simulink model "IAirHt_DD"  (R2016b)
settings: configuration reference "CodeGenConfigSet" (kept outside this file)
values from neighbouring files (symbols this model uses):
  IAirHt_stPsDiaDisbl_C = Calibration.Parameter    [init_IAirHt_DD.m]
  IAirHt_stPsDisbl_C = Calibration.Parameter    [init_IAirHt_DD.m]
  SigTst_stIAirHt_C = Calibration.Parameter    [init_IAirHt_DD.m]
  SigTst_swtIAirHt_C = Calibration.Parameter    [init_IAirHt_DD.m]
undefined symbols (not defined in the file or in its folder): Switch_conv
libraries: simulink x4
settings Model: Creator=Wei Liang  LastModifiedBy=liutao
settings ConfigSetRef: SourceLocation=Base Workspace

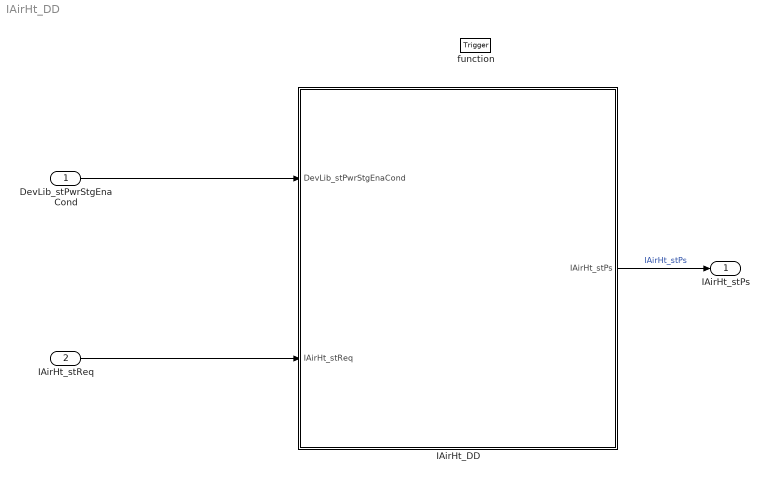
== system IAirHt_DD ==
  DevLib_stPwrStgEnaCond : Inport  Description=Control unit status relevant to power stage deactivation/error diagnosis  OutMin=0  OutMax=65535  OutDataTypeStr=State_uint16
  IAirHt_stReq : Inport  Description=Logical Output of Intake Air Heating  Port=2  OutMin=0  OutMax=1  OutDataTypeStr=boolean
  function : TriggerPort  TriggerType=function-call  VariantControl=Variant
  IAirHt_DD : Subsystem
  IAirHt_stPs : Outport  Description=Logical Output of Intake Air Heating  OutMin=0  OutMax=1  OutDataTypeStr=boolean
  wires:
  DevLib_stPwrStgEnaCond/1 -> IAirHt_DD/1(DevLib_stPwrStgEnaCond)
  IAirHt_stReq/1 -> IAirHt_DD/2(IAirHt_stReq)
  IAirHt_DD/1(IAirHt_stPs) -> IAirHt_stPs/1  "IAirHt_stPs"

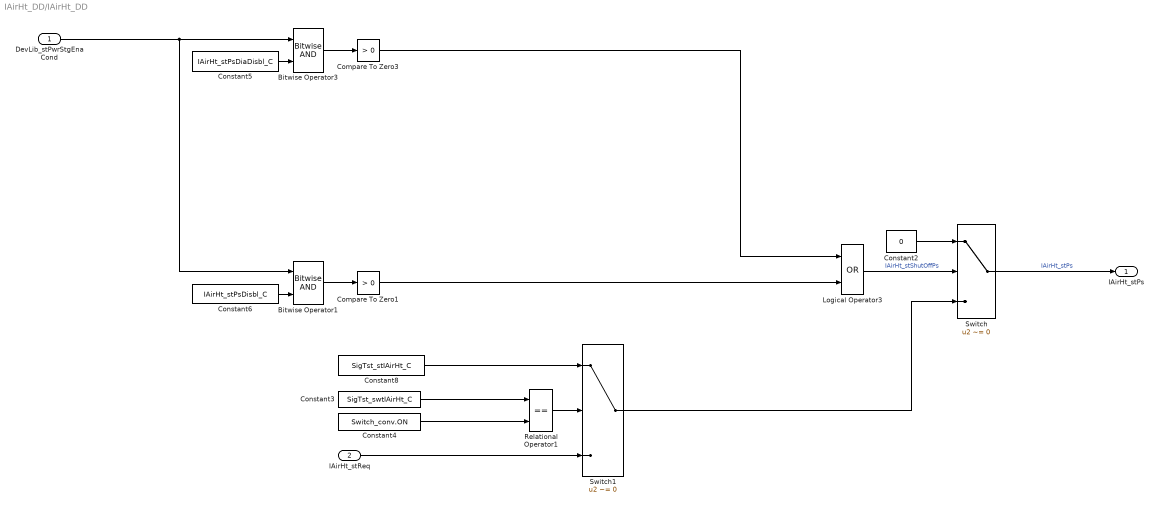
== system IAirHt_DD/IAirHt_DD ==
  DevLib_stPwrStgEnaCond : Inport  Description=Control unit status relevant to power stage deactivation/error diagnosis  OutMin=0  OutMax=65535  OutDataTypeStr=State_uint16
  IAirHt_stReq : Inport  Description=Logical Output of Intake Air Heating  Port=2  OutMin=0  OutMax=1  OutDataTypeStr=boolean
  Bitwise Operator1 : simulink/Logic and Bit Operations/Bitwise Operator  logicop=AND  UseBitMask=off  NumInputPorts=2  BitMask=bin2dec('00010000')  BitMaskRealWorld=Stored Integer
  Bitwise Operator3 : simulink/Logic and Bit Operations/Bitwise Operator  logicop=AND  UseBitMask=off  NumInputPorts=2  BitMask=bin2dec('00010000')  BitMaskRealWorld=Stored Integer
  Compare To Zero1 : simulink/Logic and Bit Operations/Compare To Zero  relop=>  OutDataTypeStr=uint8
  Compare To Zero3 : simulink/Logic and Bit Operations/Compare To Zero  relop=>  OutDataTypeStr=uint8
  Constant2 : Constant  Value=0  OutDataTypeStr=boolean  SampleTime=-1
  Constant3 : Constant  Value=SigTst_swtIAirHt_C
  Constant4 : Constant  Value=Switch_conv.ON
  Constant5 : Constant  Value=IAirHt_stPsDiaDisbl_C
  Constant6 : Constant  Value=IAirHt_stPsDisbl_C
  Constant8 : Constant  Value=SigTst_stIAirHt_C
  Logical Operator3 : Logic  Operator=OR  AllPortsSameDT=off  OutDataTypeStr=boolean
  Relational Operator1 : RelationalOperator  Operator===  OutDataTypeStr=boolean  RndMeth=Nearest
  Switch : Switch  Criteria=u2 ~= 0  SaturateOnIntegerOverflow=on  InputSameDT=on
  Switch1 : Switch  Criteria=u2 ~= 0  SaturateOnIntegerOverflow=on  InputSameDT=on
  IAirHt_stPs : Outport
  wires:
  Constant4/1 -> Relational Operator1/2
  Logical Operator3/1 -> Switch/2  "IAirHt_stShutOffPs"
  Compare To Zero1/1 -> Logical Operator3/2
  Constant2/1 -> Switch/1
  Switch/1 -> IAirHt_stPs/1  "IAirHt_stPs"
  Bitwise Operator3/1 -> Compare To Zero3/1
  Compare To Zero3/1 -> Logical Operator3/1
  DevLib_stPwrStgEnaCond/1 -> Bitwise Operator3/1, Bitwise Operator1/1
  Bitwise Operator1/1 -> Compare To Zero1/1
  Constant3/1 -> Relational Operator1/1
  Switch1/1 -> Switch/3
  Constant5/1 -> Bitwise Operator3/2
  Constant6/1 -> Bitwise Operator1/2
  IAirHt_stReq/1 -> Switch1/3
  Relational Operator1/1 -> Switch1/2
  Constant8/1 -> Switch1/1
